simulink model "TestWithDCMotor"  (R2019a)
settings: Solver=ode23  StartTime=0.0  StopTime=10.0  MaxStep=1e-2  RelTol=1e-3
undefined symbols (not defined in the file): CQ, Ke, La, Om, R, Ra, tau
libraries: simulink x1
settings Model: Creator=Bob  LastModifiedBy=Bob

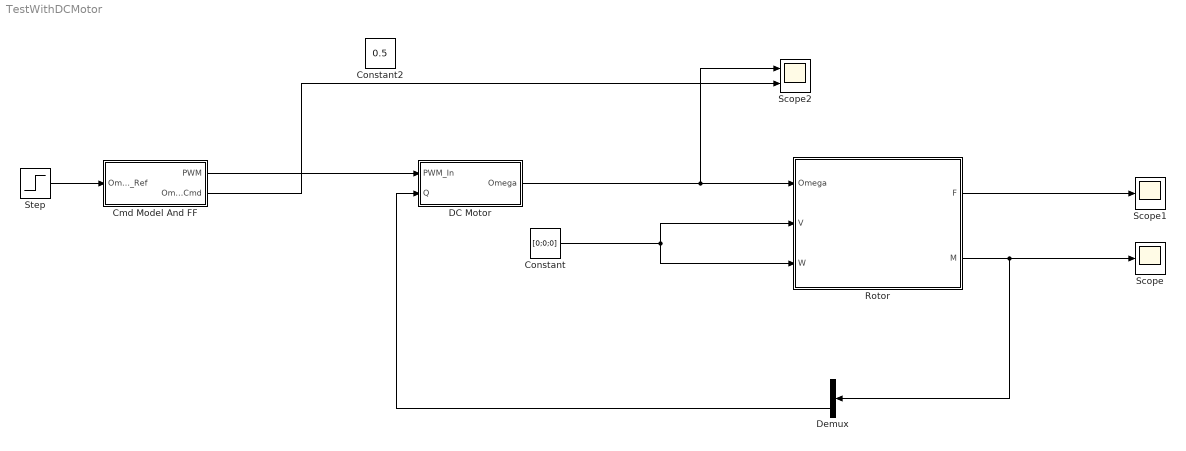
== system TestWithDCMotor ==
  Cmd Model And FF : Subsystem
  Constant : Constant  Value=[0;0;0]
  Constant2 : Constant  Value=0.5
  DC Motor : Subsystem
  Demux : Demux  Outputs=3
  Rotor : Subsystem
  Scope : Scope
  Scope1 : Scope
  Scope2 : Scope  NumInputPorts=2
  Step : Step  Time=5  Before=200  After=250  SampleTime=0
  wires:
  Constant/1 -> Rotor/3(W), Rotor/2(V)
  Rotor/2(M) -> Demux/1, Scope/1
  Rotor/1(F) -> Scope1/1
  Demux/3 -> DC Motor/2(Q)
  DC Motor/1(Omega) -> Scope2/1, Rotor/1(Omega)
  Step/1 -> Cmd Model And FF/1(Omega_Ref)
  Cmd Model And FF/1(PWM) -> DC Motor/1(PWM_In)
  Cmd Model And FF/2(Omega_Cmd) -> Scope2/2

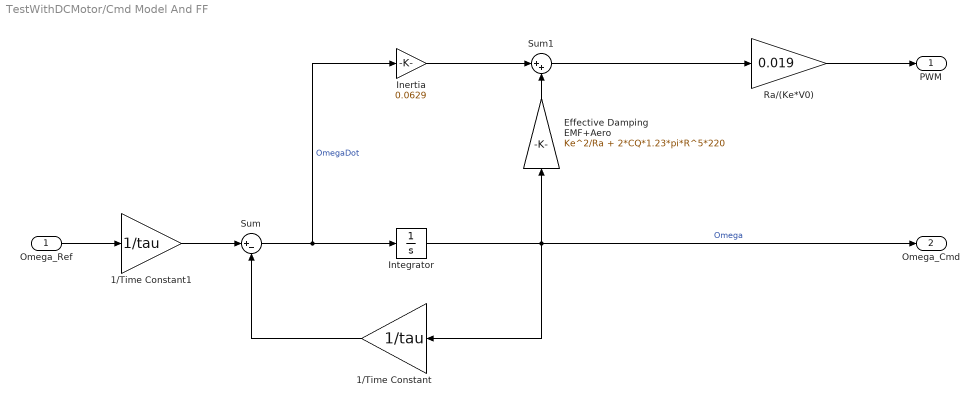
== system TestWithDCMotor/Cmd Model And FF ==
  Omega_Ref : Inport
  1/Time Constant : Gain  Gain=1/tau
  1/Time Constant1 : Gain  Gain=1/tau
  Effective Damping EMF+Aero : Gain  Gain=Ke^2/Ra + 2*CQ*1.23*pi*R^5*220
  Inertia : Gain  Gain=0.0629
  Integrator : Integrator
  Ra/(Ke*V0) : Gain  Gain=0.019
  Sum : Sum  Inputs=|+-
  Sum1 : Sum  Inputs=|++
  PWM : Outport
  Omega_Cmd : Outport  Port=2
  wires:
  Omega_Ref/1 -> 1/Time Constant1/1
  1/Time Constant1/1 -> Sum/1
  Sum/1 -> Inertia/1, Integrator/1  "OmegaDot"
  1/Time Constant/1 -> Sum/2
  Integrator/1 -> Omega_Cmd/1, Effective Damping EMF+Aero/1, 1/Time Constant/1  "Omega"
  Ra/(Ke*V0)/1 -> PWM/1
  Sum1/1 -> Ra/(Ke*V0)/1
  Effective Damping EMF+Aero/1 -> Sum1/2
  Inertia/1 -> Sum1/1

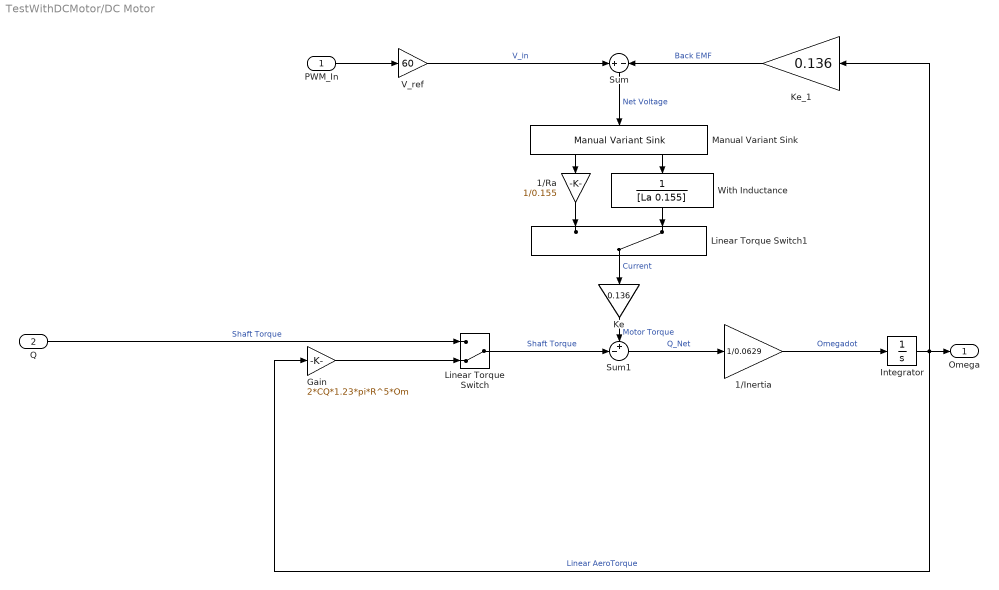
== system TestWithDCMotor/DC Motor ==
  PWM_In : Inport
  Q : Inport  Port=2
  1/Inertia : Gain  Gain=1/0.0629
  1/Ra : Gain  Gain=1/0.155
  Gain : Gain  Gain=2*CQ*1.23*pi*R^5*Om
  Integrator : Integrator
  Ke : Gain  Gain=0.136
  Ke_1 : Gain  Gain=0.136
  Linear Torque Switch : ManualSwitch  CurrentSetting=0
  Linear Torque Switch1 : ManualSwitch  CurrentSetting=0
  Manual Variant Sink : simulink/Signal Routing/Manual Variant Sink  NumChoices=2  LabelModeActiveChoice=V_2
      settings: SourceProductName=Simulink
  Sum : Sum  Inputs=+|-
  Sum1 : Sum  Inputs=+-|
  V_ref : Gain  Gain=60
  With Inductance : TransferFcn  Denominator=[La 0.155]
  Omega : Outport
  wires:
  PWM_In/1 -> V_ref/1
  V_ref/1 -> Sum/1  "V_in"
  Integrator/1 -> Gain/1, Ke_1/1, Omega/1  "Linear AeroTorque"
  1/Inertia/1 -> Integrator/1  "Omegadot"
  Ke_1/1 -> Sum/2  "Back EMF"
  Sum1/1 -> 1/Inertia/1  "Q_Net"
  Linear Torque Switch/1 -> Sum1/2  "Shaft Torque"
  Q/1 -> Linear Torque Switch/1  "Shaft Torque"
  Gain/1 -> Linear Torque Switch/2
  Sum/1 -> Manual Variant Sink/1  "Net Voltage"
  Manual Variant Sink/1 -> 1/Ra/1
  Manual Variant Sink/2 -> With Inductance/1
  1/Ra/1 -> Linear Torque Switch1/1
  With Inductance/1 -> Linear Torque Switch1/2
  Linear Torque Switch1/1 -> Ke/1  "Current"
  Ke/1 -> Sum1/1  "Motor Torque"

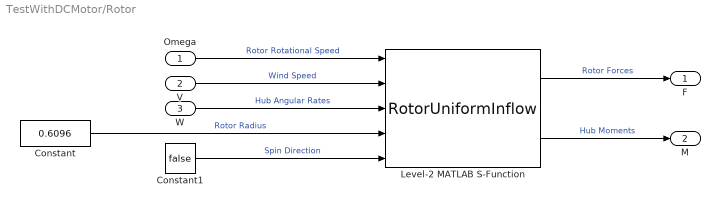
== system TestWithDCMotor/Rotor ==
  Omega : Inport  OutDataTypeStr=double
  V : Inport  Port=2  OutDataTypeStr=double
  W : Inport  Port=3  OutDataTypeStr=double
  Constant : Constant  Value=0.6096
  Constant1 : Constant  Value=false  OutDataTypeStr=boolean
  Level-2 MATLAB S-Function : M-S-Function  FunctionName=RotorUniformInflow
  F : Outport  OutDataTypeStr=double
  M : Outport  Port=2  OutDataTypeStr=double
  wires:
  Level-2 MATLAB S-Function/2 -> M/1  "Hub Moments"
  Constant/1 -> Level-2 MATLAB S-Function/4  "Rotor Radius"
  Constant1/1 -> Level-2 MATLAB S-Function/5  "Spin Direction"
  Omega/1 -> Level-2 MATLAB S-Function/1  "Rotor Rotational Speed"
  V/1 -> Level-2 MATLAB S-Function/2  "Wind Speed"
  Level-2 MATLAB S-Function/1 -> F/1  "Rotor Forces"
  W/1 -> Level-2 MATLAB S-Function/3  "Hub Angular Rates"
